simulink model "ECU2"  (R2023b)
settings: Solver=VariableStepAuto  StartTime=0.0  StopTime=Inf  RelTol=1e-3  EnableMultiTasking=on
undefined symbols (not defined in the file): canChannel
libraries: c2806xlib x8, canlib x4, canmsglib x4
settings Model: ExtModeTrigDuration=8  Creator=DELL  LastModifiedBy=DELL

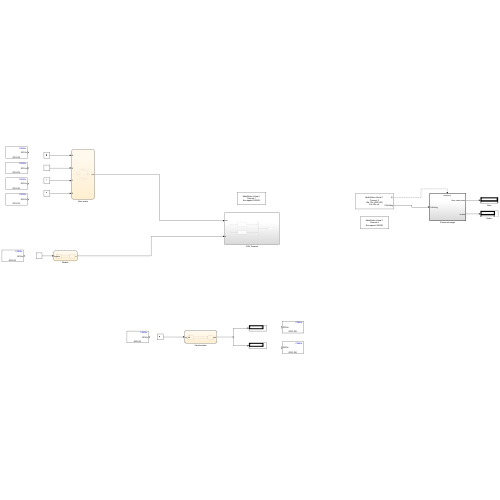
[thumbnail: Simulink's stored preview of the top-level diagram]
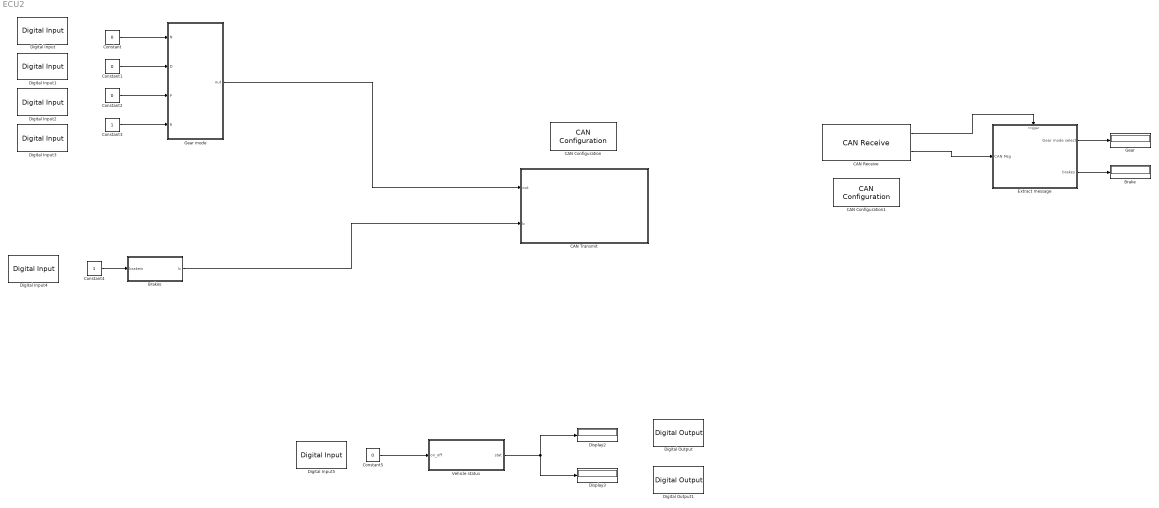
== system ECU2 ==
  Brake : Display
  Brakes : Stateflow chart  TreatAsAtomicUnit=on
  CAN Configuration : canlib/CAN Configuration  BlockHandle=13.0001  Device=MathWorks Virtual 1 (Channel 1)  DeviceMenu=MathWorks Virtual 1 (Channel 1)  ObjConstructor=canChannel('MathWorks', 'Virtual 1', 1)  BusSpeed=500000  EnableBitParameters=off  AckMode=Normal
  CAN Configuration1 : canlib/CAN Configuration  BlockHandle=14.0001  Device=MathWorks Virtual 1 (Channel 2)  DeviceMenu=MathWorks Virtual 1 (Channel 2)  ObjConstructor=canChannel('MathWorks', 'Virtual 1', 2)  BusSpeed=500000  EnableBitParameters=off  AckMode=Normal
  CAN Receive : canlib/CAN Receive  BlockHandle=15.0001  Device=MathWorks Virtual 1 (Channel 2)  DeviceMenu=MathWorks Virtual 1 (Channel 2)  ObjConstructor=canChannel('MathWorks', 'Virtual 1', 2)  EnableStandardIDsFilter=off  StdIDsCombo=Allow only  StandardIDs=[250 500]  EnableExtendedIDsFilter=off  ExtIDsCombo=Allow all  ExtendedIDs=0  SampleTime=0.01  MsgsPerTimestep=1  InternalFilterUpdateStatus=off  BusOutput=off
  CAN Transmit : Subsystem
  Constant : Constant  Value=0  OutMin=0  OutMax=8  OutDataTypeStr=uint8  LockScale=on
  Constant1 : Constant  Value=0  OutMin=0  OutMax=8  OutDataTypeStr=uint8  LockScale=on
  Constant2 : Constant  Value=0  OutMin=0  OutMax=8  OutDataTypeStr=uint8  LockScale=on
  Constant3 : Constant  OutMin=0  OutMax=8  OutDataTypeStr=uint8  LockScale=on
  Constant4 : Constant  OutMin=0  OutMax=8  OutDataTypeStr=uint8
  Constant5 : Constant  Value=0
  Digital Input : c2806xlib/Digital Input  GPIO_Number=GPIO0~GPIO7  GPIO_Bit0=on  GPIO_Bit1=off  GPIO_Bit2=off  GPIO_Bit3=off  GPIO_Bit4=off  GPIO_Bit5=off  GPIO_Bit6=off  GPIO_Bit7=off  sampleTime=0.1  dataType=auto  GPIO_Bit0_Qualification=Sync to SYSCLKOUT  GPIO_Bit1_Qualification=Sync to SYSCLKOUT  GPIO_Bit2_Qualification=Sync to SYSCLKOUT  GPIO_Bit3_Qualification=Sync to SYSCLKOUT  GPIO_Bit4_Qualification=Sync to SYSCLKOUT  GPIO_Bit5_Qualification=Sync to SYSCLKOUT  GPIO_Bit6_Qualification=Sync to SYSCLKOUT  GPIO_Bit7_Qualification=Sync to SYSCLKOUT  Qualification_Period=-1
  Digital Input1 : c2806xlib/Digital Input  GPIO_Number=GPIO0~GPIO7  GPIO_Bit0=off  GPIO_Bit1=on  GPIO_Bit2=off  GPIO_Bit3=off  GPIO_Bit4=off  GPIO_Bit5=off  GPIO_Bit6=off  GPIO_Bit7=off  sampleTime=0.1  dataType=auto  GPIO_Bit0_Qualification=Sync to SYSCLKOUT  GPIO_Bit1_Qualification=Sync to SYSCLKOUT  GPIO_Bit2_Qualification=Sync to SYSCLKOUT  GPIO_Bit3_Qualification=Sync to SYSCLKOUT  GPIO_Bit4_Qualification=Sync to SYSCLKOUT  GPIO_Bit5_Qualification=Sync to SYSCLKOUT  GPIO_Bit6_Qualification=Sync to SYSCLKOUT  GPIO_Bit7_Qualification=Sync to SYSCLKOUT  Qualification_Period=-1
  Digital Input2 : c2806xlib/Digital Input  GPIO_Number=GPIO0~GPIO7  GPIO_Bit0=off  GPIO_Bit1=off  GPIO_Bit2=on  GPIO_Bit3=off  GPIO_Bit4=off  GPIO_Bit5=off  GPIO_Bit6=off  GPIO_Bit7=off  sampleTime=0.1  dataType=auto  GPIO_Bit0_Qualification=Sync to SYSCLKOUT  GPIO_Bit1_Qualification=Sync to SYSCLKOUT  GPIO_Bit2_Qualification=Sync to SYSCLKOUT  GPIO_Bit3_Qualification=Sync to SYSCLKOUT  GPIO_Bit4_Qualification=Sync to SYSCLKOUT  GPIO_Bit5_Qualification=Sync to SYSCLKOUT  GPIO_Bit6_Qualification=Sync to SYSCLKOUT  GPIO_Bit7_Qualification=Sync to SYSCLKOUT  Qualification_Period=-1
  Digital Input3 : c2806xlib/Digital Input  GPIO_Number=GPIO0~GPIO7  GPIO_Bit0=off  GPIO_Bit1=off  GPIO_Bit2=off  GPIO_Bit3=on  GPIO_Bit4=off  GPIO_Bit5=off  GPIO_Bit6=off  GPIO_Bit7=off  sampleTime=0.1  dataType=auto  GPIO_Bit0_Qualification=Sync to SYSCLKOUT  GPIO_Bit1_Qualification=Sync to SYSCLKOUT  GPIO_Bit2_Qualification=Sync to SYSCLKOUT  GPIO_Bit3_Qualification=Sync to SYSCLKOUT  GPIO_Bit4_Qualification=Sync to SYSCLKOUT  GPIO_Bit5_Qualification=Sync to SYSCLKOUT  GPIO_Bit6_Qualification=Sync to SYSCLKOUT  GPIO_Bit7_Qualification=Sync to SYSCLKOUT  Qualification_Period=-1
  Digital Input4 : c2806xlib/Digital Input  GPIO_Number=GPIO0~GPIO7  GPIO_Bit0=off  GPIO_Bit1=off  GPIO_Bit2=off  GPIO_Bit3=off  GPIO_Bit4=on  GPIO_Bit5=off  GPIO_Bit6=off  GPIO_Bit7=off  sampleTime=0.1  dataType=auto  GPIO_Bit0_Qualification=Sync to SYSCLKOUT  GPIO_Bit1_Qualification=Sync to SYSCLKOUT  GPIO_Bit2_Qualification=Sync to SYSCLKOUT  GPIO_Bit3_Qualification=Sync to SYSCLKOUT  GPIO_Bit4_Qualification=Sync to SYSCLKOUT  GPIO_Bit5_Qualification=Sync to SYSCLKOUT  GPIO_Bit6_Qualification=Sync to SYSCLKOUT  GPIO_Bit7_Qualification=Sync to SYSCLKOUT  Qualification_Period=-1
  Digital Input5 : c2806xlib/Digital Input  GPIO_Number=GPIO0~GPIO7  GPIO_Bit0=off  GPIO_Bit1=off  GPIO_Bit2=off  GPIO_Bit3=off  GPIO_Bit4=off  GPIO_Bit5=on  GPIO_Bit6=off  GPIO_Bit7=off  sampleTime=0.1  dataType=auto  GPIO_Bit0_Qualification=Sync to SYSCLKOUT  GPIO_Bit1_Qualification=Sync to SYSCLKOUT  GPIO_Bit2_Qualification=Sync to SYSCLKOUT  GPIO_Bit3_Qualification=Sync to SYSCLKOUT  GPIO_Bit4_Qualification=Sync to SYSCLKOUT  GPIO_Bit5_Qualification=Sync to SYSCLKOUT  GPIO_Bit6_Qualification=Sync to SYSCLKOUT  GPIO_Bit7_Qualification=Sync to SYSCLKOUT  Qualification_Period=-1
  Digital Output : c2806xlib/Digital Output  GPIO_Number=GPIO0~GPIO7  GPIO_Bit0=off  GPIO_BIT0_Toggle=off  GPIO_Bit1=off  GPIO_BIT1_Toggle=off  GPIO_Bit2=off  GPIO_BIT2_Toggle=off  GPIO_Bit3=off  GPIO_BIT3_Toggle=off  GPIO_Bit4=off  GPIO_BIT4_Toggle=off  GPIO_Bit5=off  GPIO_BIT5_Toggle=off  GPIO_Bit6=on  GPIO_BIT6_Toggle=off  GPIO_Bit7=off  GPIO_BIT7_Toggle=off
  Digital Output1 : c2806xlib/Digital Output  GPIO_Number=GPIO0~GPIO7  GPIO_Bit0=off  GPIO_BIT0_Toggle=off  GPIO_Bit1=off  GPIO_BIT1_Toggle=off  GPIO_Bit2=off  GPIO_BIT2_Toggle=off  GPIO_Bit3=off  GPIO_BIT3_Toggle=off  GPIO_Bit4=off  GPIO_BIT4_Toggle=off  GPIO_Bit5=off  GPIO_BIT5_Toggle=off  GPIO_Bit6=off  GPIO_BIT6_Toggle=off  GPIO_Bit7=on  GPIO_BIT7_Toggle=off
  Display2 : Display
  Display3 : Display
  Extract message : Subsystem  TreatAsAtomicUnit=on
  Gear : Display
      settings: Format=decimal (Stored Integer)
  Gear mode : Stateflow chart  TreatAsAtomicUnit=on
  Vehicle status : Stateflow chart  TreatAsAtomicUnit=on
  wires:
  Constant/1 -> Gear mode/1(N)
  Extract message/1(Gear mode select) -> Gear/1
  CAN Receive/1 -> Extract message/Trigger
  CAN Receive/2 -> Extract message/1(CAN Msg)
  Constant1/1 -> Gear mode/2(D)
  Constant3/1 -> Gear mode/4(R)
  Constant2/1 -> Gear mode/3(P)
  Constant4/1 -> Brakes/1(brakein)
  Extract message/2(brakes) -> Brake/1
  Vehicle status/1(stat) -> Display3/1, Display2/1
  Constant5/1 -> Vehicle status/1(on_off)
  Gear mode/1(out) -> CAN Transmit/1(out)
  Brakes/1(b) -> CAN Transmit/2(b)

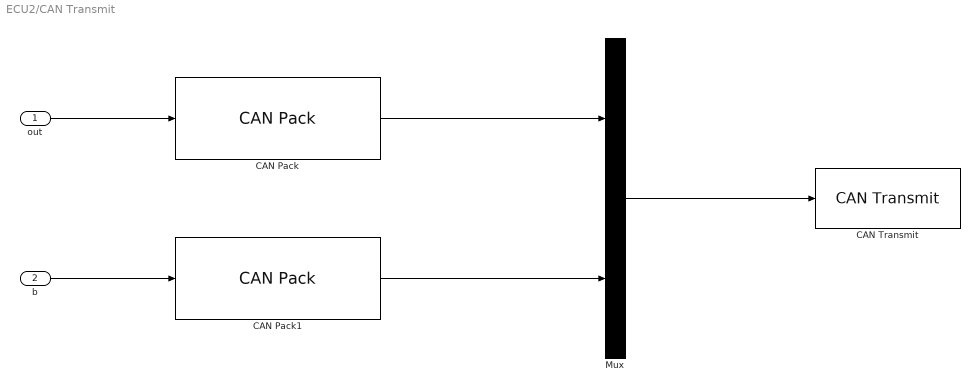
== system ECU2/CAN Transmit ==
  out : Inport
  b : Inport  Port=2
  CAN Pack : canmsglib/CAN Pack  MsgList=(none)  MsgName=CAN Msg  MsgIDType=Standard (11-bit identifier)  MsgIdentifier=250  MsgLength=8  Remote=off  ApplyMinMax=off  BusOutput=off  SignalInfo={}
      settings: LibrarySourceBlock=c2000lib/Target Communication/CAN Pack  DataFormat=raw data
  CAN Pack1 : canmsglib/CAN Pack  MsgList=(none)  MsgName=CAN Msg  MsgIDType=Standard (11-bit identifier)  MsgIdentifier=500  MsgLength=8  Remote=off  ApplyMinMax=off  BusOutput=off  SignalInfo={}
      settings: LibrarySourceBlock=c2000lib/Target Communication/CAN Pack  DataFormat=raw data
  CAN Transmit : canlib/CAN Transmit  BlockHandle=21.0001  Device=MathWorks Virtual 1 (Channel 1)  DeviceMenu=MathWorks Virtual 1 (Channel 1)  ObjConstructor=canChannel('MathWorks', 'Virtual 1', 1)  EnableEventTransmit=on  EnablePeriodicTransmit=off  MessagePeriod=1.000
  Mux : Mux  Inputs=2
  wires:
  out/1 -> CAN Pack/1
  Mux/1 -> CAN Transmit/1
  CAN Pack/1 -> Mux/1
  b/1 -> CAN Pack1/1
  CAN Pack1/1 -> Mux/2

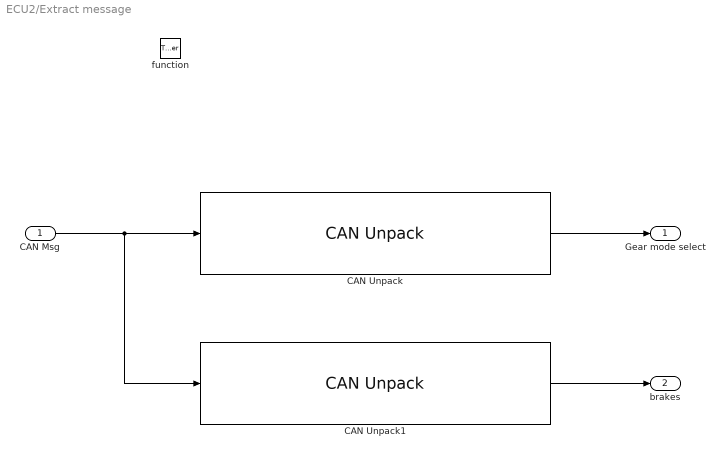
== system ECU2/Extract message ==
  CAN Msg : Inport  OutMin=0  OutMax=8  LockScale=on
  function : TriggerPort  TriggerType=function-call  VariantControl=Variant
  CAN Unpack : canmsglib/CAN Unpack  MsgList=(none)  MsgName=GearMode  MsgIDType=Standard (11-bit identifier)  MsgIdentifier=250  MsgLength=8  SignalInfo={'ThrottleCommand','0','64','LE','double','Standard','0','1','0','0','1'}  IDPort=off  TimestampPort=off  ErrorPort=off  RemotePort=off  LengthPort=off  StatusPort=off  ApplyMinMax=off
      settings: DataFormat=raw data
  CAN Unpack1 : canmsglib/CAN Unpack  MsgList=(none)  MsgName=GearMode  MsgIDType=Standard (11-bit identifier)  MsgIdentifier=500  MsgLength=8  SignalInfo={'ThrottleCommand','0','64','LE','double','Standard','0','1','0','0','1'}  IDPort=off  TimestampPort=off  ErrorPort=off  RemotePort=off  LengthPort=off  StatusPort=off  ApplyMinMax=off
      settings: DataFormat=raw data
  Gear mode select : Outport  OutMin=0  OutMax=8  OutDataTypeStr=uint8  VectorParamsAs1DForOutWhenUnconnected=off  LockScale=on
  brakes : Outport  Port=2  OutMin=0  OutMax=8  OutDataTypeStr=uint8  VectorParamsAs1DForOutWhenUnconnected=off  LockScale=on
  wires:
  CAN Msg/1 -> CAN Unpack1/1, CAN Unpack/1
  CAN Unpack/1 -> Gear mode select/1
  CAN Unpack1/1 -> brakes/1

== stateflow chart ECU2/Brakes ==
  state brakeactive
    b=1;
  state brakeinact
    b=0;
  (default) -> brakeactive
  brakeactive -> brakeinact : [brakein == 0]
  brakeinact -> brakeactive : [brakein == 1]
  data: brakein input uint8; b output uint8

== stateflow chart ECU2/Vehicle status ==
  state vehicle_off
    stat=0;
  state vehicle_on
    stat=1;
  (default) -> vehicle_off
  vehicle_off -> vehicle_on : [on_off == 1]
  vehicle_on -> vehicle_off : [on_off == 0]
  data: stat output; on_off input

== stateflow chart ECU2/Gear mode ==
  state Drive
    out=1;
  state Neutral
    out=0;
  state Reverse
    out=3;
  state Park
    out=2;
  (junction 10) -> Drive : [D == 1]
  Drive -> (junction 5) [order 3]
  Neutral -> Drive [order 3] : [D == 1]
  Drive -> Reverse [order 1] : [R == 1]
  Reverse -> Drive [order 2] : [D == 1]
  Drive -> Neutral [order 2] : [N == 1]
  Neutral -> Reverse [order 1] : [R == 1]
  (default) -> Neutral
  (junction 5) -> Park : [P == 1]
  Park -> (junction 10) [order 3]
  Reverse -> Neutral [order 1] : [N == 1]
  Park -> Neutral [order 1] : [N == 1]
  Neutral -> Park [order 2] : [P == 1]
  Reverse -> Park [order 3] : [P == 1]
  Park -> Reverse [order 2] : [R == 1]
  data: N input uint8; out output uint8; D input uint8; P input uint8; R input uint8
